simulink model "servos"  (R2024a)
settings: Solver=VariableStepAuto  StartTime=0.0  StopTime=30  RelTol=1e-3
values from neighbouring files (symbols this model uses):
  A = [-1.7, -0.25, 0 ... (first row only)    [main.m]
  B = [7, 0 ... (first row only)    [main.m]
  C = [0, 1, 0 ... (first row only)    [main.m]
  disturbance = [-2;5]    [main.m]
  K1 = K(:,1:3)    [main.m]
  K2 = K(:,4:5)    [main.m]
  L = place(A',C',desired_poles)'    [main.m]
  y_sp = [100;150]    [main.m]
settings Model: Creator=wyton  LastModifiedBy=chint
settings SolverCC: AlgebraicLoopSolver=TrustRegion
settings DebuggingCC: UnconnectedInputMsg=warning  UnconnectedOutputMsg=warning  UnconnectedLineMsg=warning
settings ModelReferenceCC: EnableRefExpFcnMdlSchedulingChecks=on
settings RTWCC: GPUComputeCapability=3.5

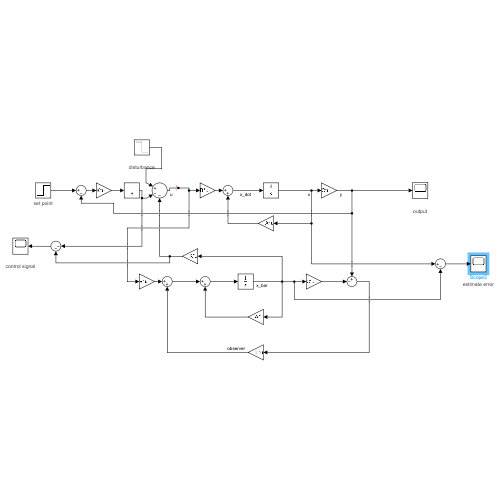
[thumbnail: Simulink's stored preview of the top-level diagram]
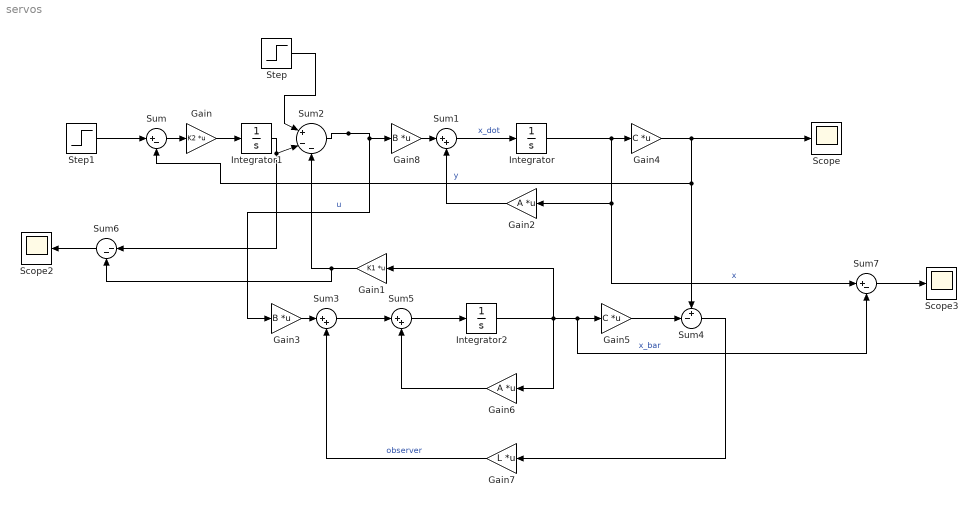
== system servos ==
  Gain : Gain  Gain=K2  Multiplication=Matrix(K*u)
  Gain1 : Gain  Gain=K1  Multiplication=Matrix(K*u)
  Gain2 : Gain  Gain=A  Multiplication=Matrix(K*u)
  Gain3 : Gain  Gain=B  Multiplication=Matrix(K*u)
  Gain4 : Gain  Gain=C  Multiplication=Matrix(K*u)
  Gain5 : Gain  Gain=C  Multiplication=Matrix(K*u)
  Gain6 : Gain  Gain=A  Multiplication=Matrix(K*u)
  Gain7 : Gain  Gain=L  Multiplication=Matrix(K*u)
  Gain8 : Gain  Gain=B  Multiplication=Matrix(K*u)
  Integrator : Integrator
  Integrator1 : Integrator
  Integrator2 : Integrator
  Scope : Scope
      settings: AttributesFormatString=output
  Scope2 : Scope
      settings: AttributesFormatString=control signal
  Scope3 : Scope
      settings: AttributesFormatString=estimate error
  Step : Step  Time=10  Before=[0;0]  After=disturbance  SampleTime=0
      settings: AttributesFormatString=disturbance
  Step1 : Step  Time=0  Before=[0;0]  After=y_sp  SampleTime=0
      settings: AttributesFormatString=set point
  Sum : Sum  Inputs=|+-
  Sum1 : Sum  Inputs=|++
  Sum2 : Sum  Inputs=|+--
  Sum3 : Sum  Inputs=|++
  Sum4 : Sum  Inputs=+-|
  Sum5 : Sum  Inputs=|++
  Sum6 : Sum  Inputs=|--
  Sum7 : Sum  Inputs=|+-
  wires:
  Sum1/1 -> Integrator/1  "x_dot"
  Gain2/1 -> Sum1/2
  Integrator/1 -> Gain2/1, Sum7/1, Gain4/1  "x"
  Gain4/1 -> Sum4/1, Sum/2, Scope/1  "y"
  Gain3/1 -> Sum3/1
  Sum3/1 -> Sum5/1
  Sum5/1 -> Integrator2/1
  Integrator2/1 -> Gain5/1, Sum7/2, Gain1/1, Gain6/1  "x_bar"
  Gain6/1 -> Sum5/2
  Gain5/1 -> Sum4/2
  Gain7/1 -> Sum3/2  "observer"
  Sum4/1 -> Gain7/1
  Gain1/1 -> Sum2/3, Sum6/2
  Gain8/1 -> Sum1/1
  Sum2/1 -> Gain8/1, Gain3/1  "u"
  Sum/1 -> Gain/1
  Gain/1 -> Integrator1/1
  Integrator1/1 -> Sum2/2, Sum6/1
  Step/1 -> Sum2/1
  Sum6/1 -> Scope2/1
  Sum7/1 -> Scope3/1
  Step1/1 -> Sum/1
